simulink model "draft2"  (R2014a)
settings: Solver=FixedStepDiscrete  StartTime=0.0  StopTime=10.0  FixedStep=1e-3  RelTol=1e-3
settings Model: Creator=Administrator  LastModifiedBy=Administrator

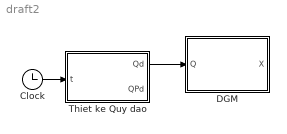
== system draft2 ==
  Clock : Clock
  DGM : MATLAB Function  TreatAsAtomicUnit=on
  Thiet ke Quy dao : MATLAB Function  TreatAsAtomicUnit=on
  wires:
  Thiet ke Quy dao/1(Qd) -> DGM/1(Q)
  Clock/1 -> Thiet ke Quy dao/1(t)

== matlab function draft2/Thiet ke Quy dao ==
  data: t input; Qd output; QPd output
function [Qd, QPd] = TKQD(t)
%#codegen
Qd = [sin(t)
      -pi/2*cos(t)];
QPd = [cos(t)
       pi/2*sin(t)];

== matlab function draft2/DGM ==
  data: Q input; X output
function X   = f(Q)
%#codegen
% Tested OK
L1 = 0.2;
L2 = 0.1442;
X1 = L1*cos(Q(1)) + L2*cos(Q(1)+Q(2));
X2 = L1*sin(Q(1)) + L2*sin(Q(1)+Q(2));
X = [X1;X2];
end
